simulink model "OASIS"  (R2024b)
settings: Solver=ode3  StartTime=0.0  StopTime=86400  FixedStep=1  MaxStep=0.1  RelTol=1e-3
PostLoadFcn:
  | init_OASIS
InitFcn:
  | init_OASIS
values from neighbouring files (symbols this model uses):
  DiscreteON = 1    [init_OASIS.m]
  GridON = 1    [init_OASIS.m]
  P_cargador_EV = 50000    [init_OASIS.m]
undefined symbols (not defined in the file or in its folder): DiscIntNeverNeededParam, Tamb
(part 1 of 3)
settings Model: PacingRate=0.500000  Creator=Miguel A. Ridao  LastModifiedBy=ferna
settings DebuggingCC: AlgebraicLoopMsg=none  UnconnectedInputMsg=warning  UnconnectedOutputMsg=warning  UnconnectedLineMsg=warning  UnderSpecifiedDimensionMsg=warning
settings ModelReferenceCC: EnableRefExpFcnMdlSchedulingChecks=on
settings RTWCC: GPUComputeCapability=3.5  DLArmComputeVersion=19.05

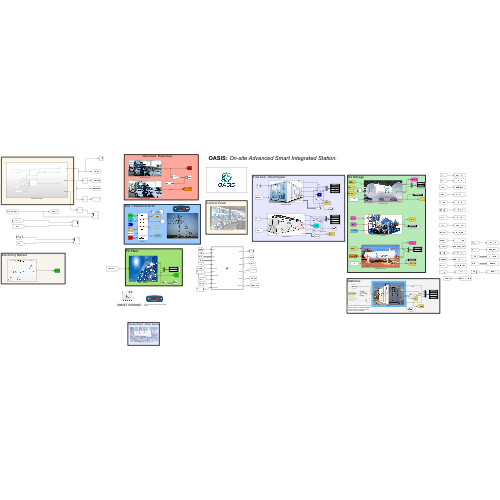
[thumbnail: Simulink's stored preview of the top-level diagram]
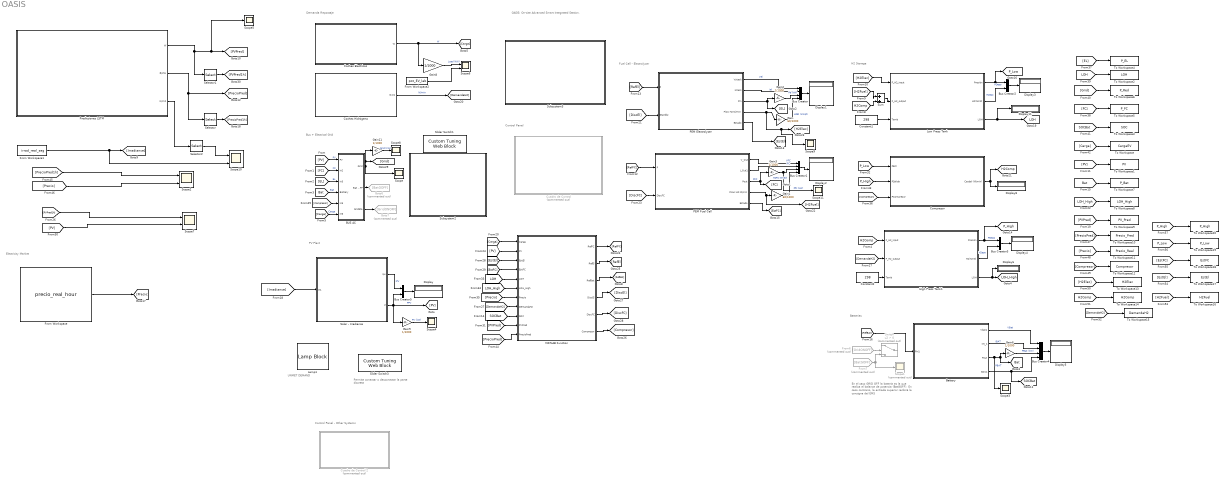
== system OASIS ==
  note: H2 Storage
  note: OASIS: On-site Advanced Smart Integrated Station.
  note: Control Panel - Other Systems
  note: En el caso GRID OFF la batería es la que realiza el balance de potencia (BatGOFF).
      | En caso contrario, la entrada superior recibirá la consigna del EMS
  note: Control Panel
  note: PV Plant
  note: Bus + Electrical Grid
  note: Demanda Repostaje
  note: Batteries
  note: Fuel Cell - Electrolyzer
  note: UNMET DEMAND
  note: Permite conectar o desconectar la parte discreta
  note: Electricity Market
  BUS AC : Subsystem
      mask Display:
      | image('Imagenes\BusAC.jpg')
      | color('red')
      | port_label('output', 1, 'Red (W)')
      | port_label('output', 2, 'Bat Grid OFF (W)')
      | port_label('output', 3, 'Grid Status')
  Battery : Subsystem  mask{Vbt0=380, CMWh=1, Kbt=0.000739, Abt=20.314, Bbt=0.00171, R=0.00027, Imax=1300, SOCact=70}
      mask prompts: Vbt0 "Open Circuit Battery Voltage, "Vbt,0" (V)"; CMWh "Maximum Capacity of the battery, "MWh)"; Kbt "Polarization Constant, "Kbt" (V)"; Abt "Amplitude of the exponential zone, "Abt" (V)"; Bbt "Inverse of the time constant in the exponencial zona, "Bbt" (A·h-1)"; R "Internal Resistance, "R" (ohms)"; Imax "Charge/Discharge Max. Current"; SOCact "SOC Initial Batteries (%)"
      mask init:
      | C120bt=CMWh*1000*1000/Vbt0
      mask DialogControl DescGroupVar Prompt: Stationary Battery model
      mask Display:
      | image('Hydor_bat.jpg')
      | color('red')
      | port_label('output', 1, 'Vbat')
      | 
      | port_label('output', 2, 'Ibat')
      | port_label('output', 3, 'Pout')
      | port_label('output', 4, 'SOC')
      | port_label('input', 1, 'P')
  Bus Creator : BusCreator  Inputs=4
  Bus Creator1 : BusCreator  Inputs=4
  Bus Creator2 : BusCreator  Inputs=2
  Bus Creator3 : BusCreator  Inputs=2
  Bus Creator4 : BusCreator  Inputs=4
  Bus Creator5 : BusCreator  Inputs=2
  Coches Electricos : Subsystem
      mask Display: image('Electric-Car.png');
  Coches Hidrógeno : Subsystem
      mask Display: image('Hydrogen_Car.png');
  Compresor : Subsystem  mask{Eficiencia=0.8, PMax=15}
      mask prompts: PMax "Potencia Máxima (kW)"
      mask Display:
      | image('Compresor.jpg'); % Use "Edit Image" on toolstrip to change.
      | color('red')
      | port_label('input', 1, 'Input Pressure [bar]')
      | port_label('input', 2, 'Output Pressure [bar]')
      | port_label('input', 3, 'Power (W)')
      | port_label('output', 1, 'H2 Flow [Nl/min]')
  Constant1 : Constant  Value=298
  Constant2 : Constant  Value=298
  Cuadro de Control : Subsystem  Commented=on
      mask Display: image('Imagenes\SCADA.jpeg')
  Cuadro de Control 2 : Subsystem  Commented=on
      mask Display: image('SCADA2.jpg'); % Use "Edit Image" on toolstrip to change.
  Display{,1..6,8,11} (9 alike) : Display
  From Workspace : FromWorkspace  VariableName=precio_real_hour  SampleTime=1  Interpolate=off  OutputAfterFinalValue=Holding final value
      mask init:
      | load('precio_horario.mat')
      mask Display: image('Imagenes\Price.PNG'); % Use "Edit Image" on toolstrip to change.
  From Workspace1 : FromWorkspace  VariableName=irrad_real_seg  SampleTime=1
  From Workspace2 : FromWorkspace  VariableName=pot_EV_lab
  From6 : From  Commented=on  GotoTag=GridONOFF
  From7 : From  Commented=on  GotoTag=BatGOFF
  Gain : Gain  Gain=60/1000
  Gain1 : Gain  Gain=60/1000
  Gain{2..3,6,8..9,11} (6 alike) : Gain  Gain=1/1000
  Goto6 : Goto  Commented=on  GotoTag=BatGOFF
  Goto7 : Goto  Commented=on  GotoTag=GridONOFF
  High Press Tank1 : Subsystem  mask{Vol=0.41, PMax=600, PIni=480}
      mask prompts: Vol "Capacidad (m3)"; PMax "Presión Máxima"; PIni "Presión Incial (bar)"
      mask Display:
      | image('Imagenes\H2DepoAlta.jpg')
      | color('red')
      | port_label('output', 1, 'Pressure [bar]')
      | port_label('output', 2, 'H2 [Nm3]')
      | port_label('output', 3, 'LOH [%]')
      | port_label('input', 1, 'H2 Elect [Nl/min]')
      | port_label('input', 2, 'H2 FC [Nl/min]')
      | port_label('input', 3, 'Temp Amb [K]')
  Lamp1 : LampBlock  LabelPosition=Hide
  Low Press Tank : Subsystem  mask{Vol=3.1, PMax=40, PIni=26}
      mask prompts: Vol "Capacidad (m3)"; PMax "Presión Máxima"; PIni "Presión Incial (bar)"
      mask Display:
      | image('Imagenes\Deposito.jpg')
      | color('red')
      | port_label('output', 1, 'Pressure [bar]')
      | port_label('output', 2, 'H2 [Nm3]')
      | port_label('output', 3, 'LOH [%]')
      | port_label('input', 1, 'H2 Elect [Nl/min]')
      | port_label('input', 2, 'H2 FC [Nl/min]')
      | port_label('input', 3, 'Temp Amb [K]')
  MATLAB Function : MATLAB Function  TreatAsAtomicUnit=on
  PEM Electrolyser : Subsystem  mask{E0=1.23, K1n=-0.9e-3, Ph2=40, Po2=1.3, Ael=1500, Rohm=1.7008e-04, iao=1.0631e-6, ico=1e-3, N=60, Tel=298, Pmax=200000, Pout=40, efc=0.7, efcv=0.97}
      mask prompts: E0 "E0 (V)"; Ph2 "Hydrogen Partial Pressure (bar)"; Po2 "Oxygen Partial Pressure (bar)"; Ael "Stack Area (cm^2)"; iao "Anode Current Density (A/cm^2)"; ico "Cathode Current Density (A/cm^2)"; N "Number of Cells in the Stack"; Tel "Electrolizer Temperature (K)"; Pmax "Max Input Power (W)"; Pout "Tank pressure (bar)"; efc "Compressor Efficiency"; efcv "Converter Efficiancy"
      mask init:
      | R=8.314472;
      | F=96485;
      | CpH2=20.79;
      | gamma=1.4;
      | 
      | ModoManual=1;
      | PElecMan=100;
      mask Help:
      | INPUTS
      | - Power (W)  Power hss to be negative
      | 
      | OUTPUTS
      | - Electrolizer Voltage (V)
      | - Electrolizar Current (I)
      | - H2 Flow (g/s)
      mask DialogControl DescGroupVar Prompt: PEM Electrolyser Model
      mask DialogControl DescTextVar Prompt: (Add text here)
      mask DialogControl ParameterGroupVar Prompt: PEM Electrolyser Parameters
      mask Display:
      | image('Hydor_elec.jpg')
      | color('red')
      | port_label('output', 1, 'Vel')
      | port_label('output', 2, 'Iel')
      | port_label('output', 4, 'H2 (Nl/min)')
      | port_label('output', 5, 'Estado')
      | port_label('output', 3, 'Pin')
      | port_label('input', 1, 'P')
  PEM Fuel Cell : Subsystem  mask{u0=0.93, K1t=0.00293, K1act=0.066098, K2act=0.012705, Rohm=0.29179, K1conc=0.028396, K2conc=8.0011, Tst=296, T0st=296, Afc=600, n=120, Imax=600}
      mask prompts: Tst "Stack Temperature (K)"; T0st "Nominal Stack Temperature (K)"; Afc "Effective Area of the Membrane (cm^2)"; n "Number of Cell in the Fuel Cell"; Imax "Max Corrent (A)"
      mask init:
      | R=8.314472;
      | F=96485;
      mask DialogControl DescGroupVar Prompt: Fuell Cell Model
      mask DialogControl ParameterGroupVar Prompt: Equation Parameters
      mask DialogControl Container4 Prompt: Fuel Cell Parameters
      mask Display:
      | image('Imagenes\Hydor_FC.jpg')
      | color('red')
      | port_label('output', 1, 'Vst')
      | 
      | 
      | port_label('input', 1, 'P')
      | 
      | port_label('output', 3, 'Pout')
      | 
      | port_label('output', 2, 'Ist')
      | port_label('output', 4, 'H2 (Nl/min)')
      | port_label('output', 5, 'Estado')
  Predicciones LSTM : Subsystem
  Scope{,3..5,8..9,11} (7 alike) : Scope
  Scope1 : Scope  Commented=on
  Scope{2,6..7,10} (4 alike) : Scope  NumInputPorts=2
  Selector : Selector  InputPortWidth=24  IndexOptions=Index vector (dialog)  Indices=[1]  OutputSizes=1
  Selector1 : Selector  InputPortWidth=24  IndexOptions=Index vector (dialog)  Indices=[1]  OutputSizes=1
  Selector2 : Selector  InputPortWidth=24  IndexOptions=Index vector (dialog)  Indices=[1]  OutputSizes=1
  Slider Switch1 : CustomTuningWebBlock  LabelPosition=Hide  ShowInitialText=on  Configuration="{\"components\":[{\"name\":\"CustomSwitchStateComponent\",\"settings\":{\"position\":[0,0,1,1],\"states\":[{\"HitRegion\":{\"position\":[0,0,0.5,1]},\"Image\":{\"position\":[0,0,1,1],\"size\":[1,1],\"src\":\"data:image\\/svg+xml;base64,PD94bWwgdmVyc2lvbj0iMS4wIiBlbmNvZGluZz0idXRmLTgiPz4NCjwhLS0gR2VuZXJhdG9yOiBBZG9iZSBJbGx1c3RyYXRvciAyNS4yLjEsIFNWRyBFeHBvcnQgUGx1Zy1JbiAuIFNWRyBWZXJzaW9uOiA2LjAwIEJ1aWxkIDApICAtLT4NCjxzdmcgdmVyc2lvbj0iMS4xIiB4bWxucz0iaHR0cDovL3d3dy53My5vcmcvMjAwMC9zdmciIHhtbG5zOnhsaW5rPSJodHRwOi8vd3d3LnczLm9yZy8xOTk5L3hsaW5rIiB4PSIwcHgiIHk9IjBweCINCgkgdmlld0JveD0iMCAwIDc2IDI5IiBzdHlsZT0iZW5hYmxlLWJhY2tncm91bmQ6bmV3 ...(+5404 chars)\",\"srcOrientation\":\"Right\"},\"Label\":{\"color\":[0.9882352941176471,0.9882352941176471,0.7725490196078432],\"icon\":{\"size\":[0,0],\"src\":[],\"srcOrientation\":\"Right\"},\"iconPlacement\":\"left\",\"opacity\":1,\"position\":[0.5,0.14],\"show\":true,\"text\":{\"content\":\"Off\",\"font\":\"Helvetica\"}},\"Value\":0},{\"HitRegion\":{\"position\":[0,0.5,0.5,1]},\"Image\":{\"position\":[0,0,1,1],\"size\":[1,1],\"src\":\"data:image\\/svg+xml;base64,PD94bWwgdmVyc2lvbj0iMS4wIiBlbmNvZGluZz0idXRmLTgiPz4NCjwhLS0gR2VuZXJhdG9yOiBBZG9iZSBJbGx1c3RyYXRvciAyNS4yLjEsIFNWRyBFeHBvcnQgUGx1Zy1JbiAuIFNWRyBWZXJzaW9uOiA2LjAwIEJ1aWxkIDApICAtLT4NCjxzdmcgdmVyc2lvbj0iMS4xIiB4bWxucz0iaHR0cDovL3d3dy53My5vcmcvMjAwMC9zdmciIHhtbG5zOnhsaW5rPSJodHRwOi8vd3d3LnczLm9yZy8xOTk5L3hsaW5rIiB4PSIwcHgiIHk9IjBweCINCgkgdmlld0JveD0iMCAwIDc2IDI5IiBzdHlsZT0iZW5hYmxlLWJhY2tncm91bmQ6bmV3 ...(+5404 chars)\",\"srcOrientation\":\"Right\"},\"Label\":{\"color\":[0.9882352941176471,0.9882352941176471,0.7725490196078432],\"icon\":{\"size\":[0,0],\"src\":[],\"srcOrientation\":\"Right\"},\"iconPlacement\":\"left\",\"opacity\":1,\"position\":[0.5,0.86],\"show\":true,\"text\":{\"content\":\"On\",\"font\":\"Helvetica\"}},\"Value\":1}]}},{\"name\":\"BackgroundImageComponent\",\"settings\":{\"image\":{\"size\":[0,0],\"src\":\"default\",\"srcOrientation\":[]},\"position\":[0,0,1,1],\"scaleMode\":\"0\"}},{\"name\":\"ForegroundImageComponent\",\"settings\":{\"image\":{\"size\":[0,0],\"src\":\"default\",\"srcOrientation\":[]},\"isForeground\":1,\"position\":[0,0,1,1],\"scaleMode\":\"0\"}}],\"settings\":{\"BindingType\":\"param\",\"backgroundColor\":[0,0,255,\"1\"],\"fixedAspectRatio\":\"on\",\"foregroundColor\":[234,234,234],\"showBackgroundColor\":false,\"variant\":\"slider\",\"version\":\"R2024b\"},\"type\":\"Switch\"}"
  Slider Switch3 : CustomTuningWebBlock  LabelPosition=Hide  ShowInitialText=on  Configuration="{\"components\":[{\"name\":\"CustomSwitchStateComponent\",\"settings\":{\"position\":[0,0,1,1],\"states\":[{\"HitRegion\":{\"position\":[0,0,0.5,1]},\"Image\":{\"position\":[0,0,1,1],\"size\":[1,1],\"src\":\"data:image\\/svg+xml;base64,PD94bWwgdmVyc2lvbj0iMS4wIiBlbmNvZGluZz0idXRmLTgiPz4NCjwhLS0gR2VuZXJhdG9yOiBBZG9iZSBJbGx1c3RyYXRvciAyNS4yLjEsIFNWRyBFeHBvcnQgUGx1Zy1JbiAuIFNWRyBWZXJzaW9uOiA2LjAwIEJ1aWxkIDApICAtLT4NCjxzdmcgdmVyc2lvbj0iMS4xIiB4bWxucz0iaHR0cDovL3d3dy53My5vcmcvMjAwMC9zdmciIHhtbG5zOnhsaW5rPSJodHRwOi8vd3d3LnczLm9yZy8xOTk5L3hsaW5rIiB4PSIwcHgiIHk9IjBweCINCgkgdmlld0JveD0iMCAwIDc2IDI5IiBzdHlsZT0iZW5hYmxlLWJhY2tncm91bmQ6bmV3 ...(+5404 chars)\",\"srcOrientation\":\"Right\"},\"Label\":{\"color\":[0.9882352941176471,0.9882352941176471,0.7725490196078432],\"icon\":{\"size\":[0,0],\"src\":[],\"srcOrientation\":\"Right\"},\"iconPlacement\":\"left\",\"opacity\":1,\"position\":[0.5,0.14],\"show\":true,\"text\":{\"content\":\"Off\",\"font\":\"Helvetica\"}},\"Value\":0},{\"HitRegion\":{\"position\":[0,0.5,0.5,1]},\"Image\":{\"position\":[0,0,1,1],\"size\":[1,1],\"src\":\"data:image\\/svg+xml;base64,PD94bWwgdmVyc2lvbj0iMS4wIiBlbmNvZGluZz0idXRmLTgiPz4NCjwhLS0gR2VuZXJhdG9yOiBBZG9iZSBJbGx1c3RyYXRvciAyNS4yLjEsIFNWRyBFeHBvcnQgUGx1Zy1JbiAuIFNWRyBWZXJzaW9uOiA2LjAwIEJ1aWxkIDApICAtLT4NCjxzdmcgdmVyc2lvbj0iMS4xIiB4bWxucz0iaHR0cDovL3d3dy53My5vcmcvMjAwMC9zdmciIHhtbG5zOnhsaW5rPSJodHRwOi8vd3d3LnczLm9yZy8xOTk5L3hsaW5rIiB4PSIwcHgiIHk9IjBweCINCgkgdmlld0JveD0iMCAwIDc2IDI5IiBzdHlsZT0iZW5hYmxlLWJhY2tncm91bmQ6bmV3 ...(+5404 chars)\",\"srcOrientation\":\"Right\"},\"Label\":{\"color\":[0.9882352941176471,0.9882352941176471,0.7725490196078432],\"icon\":{\"size\":[0,0],\"src\":[],\"srcOrientation\":\"Right\"},\"iconPlacement\":\"left\",\"opacity\":1,\"position\":[0.5,0.86],\"show\":true,\"text\":{\"content\":\"On\",\"font\":\"Helvetica\"}},\"Value\":1}]}},{\"name\":\"BackgroundImageComponent\",\"settings\":{\"image\":{\"size\":[0,0],\"src\":\"default\",\"srcOrientation\":[]},\"position\":[0,0,1,1],\"scaleMode\":\"0\"}},{\"name\":\"ForegroundImageComponent\",\"settings\":{\"image\":{\"size\":[0,0],\"src\":\"default\",\"srcOrientation\":[]},\"isForeground\":1,\"position\":[0,0,1,1],\"scaleMode\":\"0\"}}],\"settings\":{\"BindingType\":\"param\",\"backgroundColor\":[0,0,255,\"1\"],\"fixedAspectRatio\":\"on\",\"foregroundColor\":[234,234,234],\"showBackgroundColor\":false,\"variant\":\"slider\",\"version\":\"R2024b\"},\"type\":\"Switch\"}"
  Solar - Irradiance : Subsystem  mask{npar=35, nser=24, Vp=34.60, Isc=18.57, Voc=41.7, Tc=300}
      mask prompts: npar "Number of modules in parallel"; nser "Number of modules in serie"; Vp "Voltage in the Maximun Power Point (V)"; Isc "Short Circuit Current (A)"; Voc "Open circuit Voltage (V)"; Tc "Temperature (K)"
      mask init:
      | % electron charge
      | e=1.6e-19;%(C)
      | %Boltzman constant
      | k=1.381e-23;%(J/K)
      | %Serial Resistor
      | Rs=0.1;
      mask DialogControl DescGroupVar Prompt: Photovoltaic Cell Model
      mask Display:
      | image('Imagenes\sun.jpg')
      | color('red')
      | port_label('output', 1, 'Ipv')
      | port_label('output', 2, 'Psf')
  Subsystem2 : Subsystem
      mask Display: image('Red.jpeg'); % Use "Edit Image" on toolstrip to change.
  Subsystem3 : Subsystem
      mask Display: image('OASIS.png');
  Sum : Sum  Inputs=|++
  Switch : Switch  Commented=on  Criteria=u2 > Threshold  SaturateOnIntegerOverflow=off  InputSameDT=off
  To Workspace : ToWorkspace  VariableName=CargaEV  SaveFormat=Timeseries  SampleTime=-1
  To Workspace1 : ToWorkspace  VariableName=PV  SaveFormat=Timeseries  SampleTime=-1
  To Workspace10 : ToWorkspace  VariableName=Precio_Pred  SaveFormat=Timeseries  SampleTime=-1
  To Workspace11 : ToWorkspace  VariableName=Precio_Real  SaveFormat=Timeseries  SampleTime=-1
  To Workspace12 : ToWorkspace  VariableName=Compresor  SaveFormat=Timeseries  SampleTime=-1
  To Workspace13 : ToWorkspace  VariableName=H2Elec  SaveFormat=Timeseries  SampleTime=-1
  To Workspace14 : ToWorkspace  VariableName=H2Comp  SaveFormat=Timeseries  SampleTime=-1
  To Workspace15 : ToWorkspace  VariableName=DemandaH2  SaveFormat=Timeseries  SampleTime=-1
  To Workspace16 : ToWorkspace  VariableName=H2Fuel  SaveFormat=Timeseries  SampleTime=-1
  To Workspace17 : ToWorkspace  VariableName=EstEl  SaveFormat=Timeseries  SampleTime=-1
  To Workspace18 : ToWorkspace  VariableName=EstFC  SaveFormat=Timeseries  SampleTime=-1
  To Workspace19 : ToWorkspace  VariableName=P_Low  SaveFormat=Timeseries  SampleTime=-1
  To Workspace2 : ToWorkspace  VariableName=LOH  SaveFormat=Timeseries  SampleTime=-1
  To Workspace20 : ToWorkspace  VariableName=P_High  SaveFormat=Timeseries  SampleTime=-1
  To Workspace3 : ToWorkspace  VariableName=SOC  SaveFormat=Timeseries  SampleTime=-1
  To Workspace4 : ToWorkspace  VariableName=P_EL  SaveFormat=Timeseries  SampleTime=-1
  To Workspace5 : ToWorkspace  VariableName=P_FC  SaveFormat=Timeseries  SampleTime=-1
  To Workspace6 : ToWorkspace  VariableName=P_Red  SaveFormat=Timeseries  SampleTime=-1
  To Workspace7 : ToWorkspace  VariableName=P_Bat  SaveFormat=Timeseries  SampleTime=-1
  To Workspace8 : ToWorkspace  VariableName=LOH_High  SaveFormat=Timeseries  SampleTime=-1
  To Workspace9 : ToWorkspace  VariableName=PV_Pred  SaveFormat=Timeseries  SampleTime=-1
  tag scope: Bat=global, H2Comp=global, LOH=global, LOH_High=global, P_High=global, P_Low=global, SOCBat=global
  wires:
  Solar - Irradiance/1(Ipv) -> Bus Creator5/1  "IPV"
  PEM Electrolyser/1(Vstack) -> Bus Creator/1  "Vel"
  PEM Electrolyser/2(Istack) -> Bus Creator/2  "Iel"
  PEM Electrolyser/3(Pin) -> Gain2/1, [EL]
  PEM Electrolyser/4("Flow H2 Nl/min ") -> Scope9/1, [H2Elec], Gain/1
  Low Press Tank/1(Presión) -> [P_Low], Bus Creator2/1  "PDepo"
  Low Press Tank/2(H2(Nm3)) -> Bus Creator2/2  "H2epo"
  Constant1/1 -> Low Press Tank/3(Tamb)
  Gain/1 -> Bus Creator/4  "H2El  Nm3/h"
  PEM Fuel Cell/1(V_Out) -> Bus Creator1/1  "VFC"
  PEM Fuel Cell/3(Pout) -> Gain3/1, [FC]  "PFC"
  PEM Fuel Cell/4(Flowl H2 Nl/min) -> [H2Fuel], Gain1/1
  Gain1/1 -> Bus Creator1/4  "H2FC Nm3/h"
  Battery/2(Int_1) -> Bus Creator4/2  "IBAT"
  Battery/4(SOC1) -> [SOCBat], Bus Creator4/4
  Coches Electricos/1(W) -> Gain8/1, [Carga]  "W"
  [PV] -> BUS AC/1(PV)  "PV"
  [FC] -> BUS AC/2(In2)  "FC"
  [EL] -> BUS AC/3(In3)  "EL"
  [Bat] -> BUS AC/4(Battery)  "Bat"
  [Carga] -> BUS AC/6(In6)  "Carga"
  PEM Fuel Cell/2(I_Out1) -> Bus Creator1/2  "IFC"
  Bus Creator/1 -> Display1/1
  Gain2/1 -> Bus Creator/3  "Pe (kW)"
  Bus Creator1/1 -> Display2/1
  Bus Creator2/1 -> Display3/1
  Battery/1(Vbat1) -> Bus Creator4/1  "VBat"
  Battery/3(Pout) -> Scope3/1, Gain6/1, [Bat]  "PBAT"
  Bus Creator4/1 -> Display5/1
  Solar - Irradiance/2(P) -> [PV], Gain9/1, Bus Creator5/2  "PPV"
  Bus Creator5/1 -> Display/1
  Gain3/1 -> Scope11/1, Bus Creator1/3  "Pfc (kW)"
  BUS AC/1(Grid) -> Scope/1, Gain11/1, [Grid]
  BUS AC/2(Bat GOFF) -> Goto6/1
  BUS AC/3(GridSta) -> Goto7/1
  From6/1 -> Switch/2
  From7/1 -> Scope1/1, Switch/3
  Gain6/1 -> Bus Creator4/3  "PBat (kW)"
  [RefFC] -> PEM Fuel Cell/1(P)
  [RefEl] -> PEM Electrolyser/1(P)
  Gain8/1 -> Scope6/1  "Load (kW)"
  Gain9/1 -> Scope4/1  "PV (kW)"
  Gain11/1 -> Scope8/1  "Grid (kW)"
  PEM Electrolyser/5(Estado) -> [EstEl]
  [DiscEl] -> PEM Electrolyser/2(Standby)
  PEM Fuel Cell/5(Estado) -> [EstFC]
  [DiscFC] -> PEM Fuel Cell/2(DiscFC)
  Low Press Tank/3(LOH) -> Display11/1, [LOH]
  [RefBat] -> Battery/1(Pin1)
  Constant2/1 -> High Press Tank1/3(Tamb)
  High Press Tank1/3(LOH) -> Display6/1, [LOH_High]
  Bus Creator3/1 -> Display4/1
  High Press Tank1/1(Presión) -> [P_High], Bus Creator3/1  "PDepo"
  High Press Tank1/2(H2(Nm3)) -> Bus Creator3/2  "H2epo"
  [P_Low] -> Compresor/1(PEnt)
  [P_High] -> Compresor/2(PSalida)
  Compresor/1(Caudal (Nl/min)) -> [H2Comp], Display8/1
  [H2Comp] -> High Press Tank1/1(F_H2_input)
  Sum/1 -> Low Press Tank/2(F_H2_output)
  [H2Fuel] -> Sum/1
  [H2Comp] -> Sum/2
  [H2Elec] -> Low Press Tank/1(F_H2_input)
  [DemandaH2] -> High Press Tank1/2(F_H2_output)
  [Carga] -> MATLAB Function/1(Carga)
  [PV] -> MATLAB Function/2(PV)
  [EstEl] -> MATLAB Function/3(EstEl)
  [EstFC] -> MATLAB Function/4(EstFC)
  [LOH] -> MATLAB Function/5(LOH)
  [LOH_High] -> MATLAB Function/6(LOH_High)
  [Precio] -> MATLAB Function/7(Precio)
  MATLAB Function/1(RefFC) -> [RefFC]
  MATLAB Function/2(RefEl) -> [RefEl]
  MATLAB Function/4(DiscEl) -> [DiscEl]
  MATLAB Function/5(DiscFC) -> [DiscFC]
  [DemandaH2] -> MATLAB Function/8(DemandaH2)
  [Compresor] -> Compresor/3(PCompresor)
  MATLAB Function/6(Compresor) -> [Compresor]
  Coches Hidrógeno/1(Out1) -> [DemandaH2]  "Nl/min"
  [EL] -> To Workspace4/1
  [FC] -> To Workspace5/1
  [LOH] -> To Workspace2/1
  [Grid] -> To Workspace6/1
  [SOCBat] -> To Workspace3/1
  [Carga] -> To Workspace/1
  [PV] -> To Workspace1/1
  [SOCBat] -> MATLAB Function/9(SOC)
  MATLAB Function/3(RefBat) -> [RefBat]
  [Bat] -> To Workspace7/1
  [LOH_High] -> To Workspace8/1
  [Compresor] -> BUS AC/5(In5)
  From Workspace1/1 -> Scope10/2, [Irradiance]
  [Irradiance] -> Solar - Irradiance/1(In1)
  [PVPred] -> To Workspace9/1
  [PV] -> Scope7/2
  [PVPred1h] -> Scope7/1
  [PVPred] -> MATLAB Function/10(PVPred)
  From Workspace/1 -> [Precio]
  Predicciones LSTM/1(W) -> Selector1/1, Scope5/1, [PVPred]
  Predicciones LSTM/2(€/MW) -> Selector/1, [PrecioPred]
  [Precio] -> Scope2/2
  [PrecioPred1h] -> Scope2/1
  Selector/1 -> [PrecioPred1h]
  Selector1/1 -> [PVPred1h]
  [PrecioPred] -> MATLAB Function/11(PrecioPred)
  Predicciones LSTM/3(W/m2) -> Selector2/1
  Selector2/1 -> Scope10/1
  [PrecioPred] -> To Workspace10/1
  [Precio] -> To Workspace11/1
  From Workspace2/1 -> Scope6/2
  [Compresor] -> To Workspace12/1
  [H2Elec] -> To Workspace13/1
  [H2Comp] -> To Workspace14/1
  [DemandaH2] -> To Workspace15/1
  [H2Fuel] -> To Workspace16/1
  [EstEl] -> To Workspace17/1
  [EstFC] -> To Workspace18/1
  [P_Low] -> To Workspace19/1
  [P_High] -> To Workspace20/1

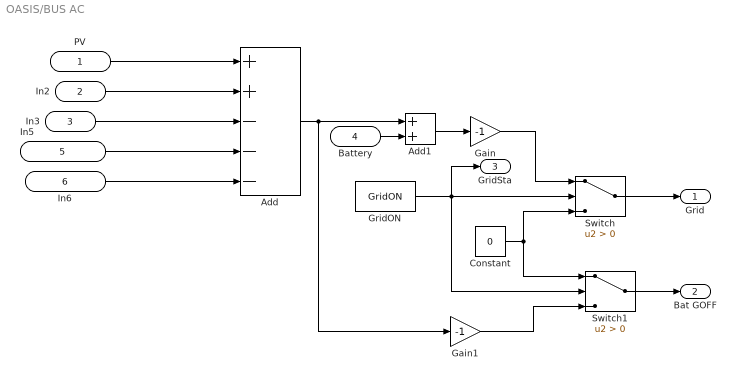
== system OASIS/BUS AC ==
  PV : Inport
  In2 : Inport  Port=2
  In3 : Inport  Port=3
  Battery : Inport  Port=4
  In5 : Inport  Port=5
  In6 : Inport  Port=6
  Add : Sum  Inputs=++---
  Add1 : Sum
  Constant : Constant  Value=0
  Gain : Gain  Gain=-1
  Gain1 : Gain  Gain=-1
  GridON : Constant  Value=GridON
  Switch : Switch  Criteria=u2 > Threshold  SaturateOnIntegerOverflow=off  InputSameDT=off
  Switch1 : Switch  Criteria=u2 > Threshold  SaturateOnIntegerOverflow=off  InputSameDT=off
  Grid : Outport
  Bat GOFF : Outport  Port=2
  GridSta : Outport  Port=3
  wires:
  GridON/1 -> GridSta/1, Switch/2, Switch1/2
  PV/1 -> Add/1
  In2/1 -> Add/2
  In3/1 -> Add/3
  In6/1 -> Add/5
  Add/1 -> Gain1/1, Add1/1
  Battery/1 -> Add1/2
  Add1/1 -> Gain/1
  Gain/1 -> Switch/1
  Switch/1 -> Grid/1
  Constant/1 -> Switch/3, Switch1/1
  Switch1/1 -> Bat GOFF/1
  Gain1/1 -> Switch1/3
  In5/1 -> Add/4

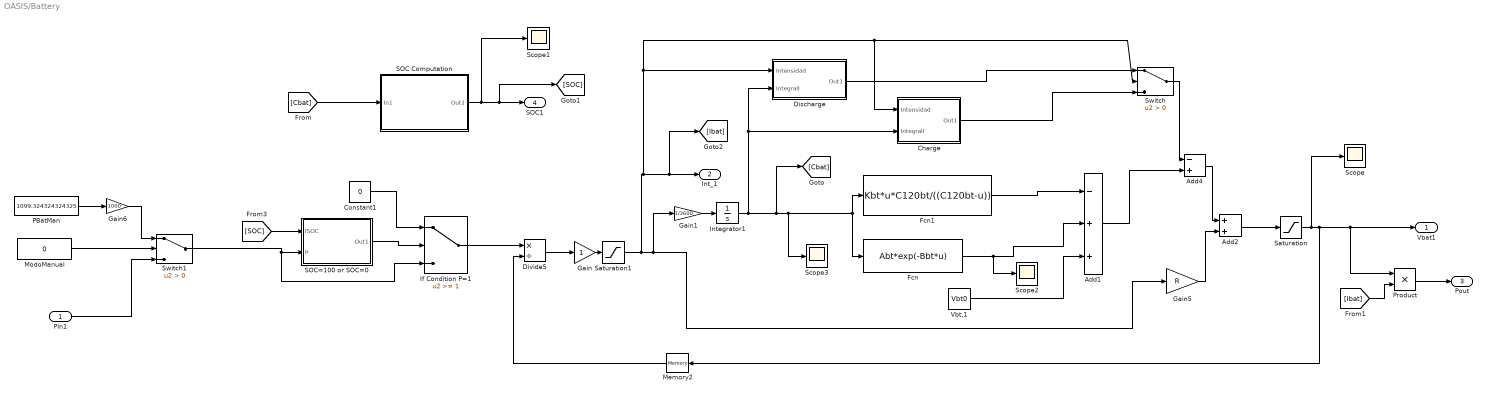
== system OASIS/Battery ==
  Pin1 : Inport
  Add1 : Sum  Inputs=-++
  Add2 : Sum
  Add4 : Sum  Inputs=-+
  Charge : Subsystem
  Constant1 : Constant  Value=0
  Discharge : Subsystem
  Divide5 : Product  Inputs=*/
  Fcn : Fcn  Expr=Abt*exp(-Bbt*u)
  Fcn1 : Fcn  Expr=Kbt*u*C120bt/((C120bt-u))
  Gain : Gain
  Gain1 : Gain  Gain=1/3600
  Gain5 : Gain  Gain=R
  Gain6 : Gain  Gain=1000
  If Condition P=1 : Switch  Threshold=1  SaturateOnIntegerOverflow=off  InputSameDT=off
  Integrator1 : Integrator  InitialCondition=C120bt-(SOCact/100)*C120bt  LimitOutput=on  UpperSaturationLimit=C120bt  LowerSaturationLimit=0
  Memory2 : Memory  InitialCondition=48
  ModoManual : Constant  Value=0
  PBatMan : Constant  Value=1099.324324324325
  Product : Product
  SOC Computation : Subsystem
  SOC=100 or SOC=0 : Subsystem
  Saturation : Saturate  UpperLimit=inf  LowerLimit=1
  Saturation1 : Saturate  UpperLimit=Imax  LowerLimit=-Imax
  Scope{,1..3} (4 alike) : Scope
  Switch : Switch  Criteria=u2 > Threshold  SaturateOnIntegerOverflow=off  InputSameDT=off
  Switch1 : Switch  Criteria=u2 > Threshold  SaturateOnIntegerOverflow=off  InputSameDT=off
  Vbt,1 : Constant  Value=Vbt0
  Vbat1 : Outport  VectorParamsAs1DForOutWhenUnconnected=off
  Int_1 : Outport  Port=2  VectorParamsAs1DForOutWhenUnconnected=off
  Pout : Outport  Port=3  VectorParamsAs1DForOutWhenUnconnected=off
  SOC1 : Outport  Port=4  VectorParamsAs1DForOutWhenUnconnected=off
  wires:
  ModoManual/1 -> Switch1/2
  Pin1/1 -> Switch1/3
  Gain6/1 -> Switch1/1
  PBatMan/1 -> Gain6/1
  [Ibat] -> Product/2
  SOC=100 or SOC=0/1(Out1) -> If Condition P=1/2
  [Cbat] -> SOC Computation/1(In1)
  Saturation/1 -> Scope/1, Memory2/1, Vbat1/1, Product/1
  Integrator1/1 -> Charge/2(IntegralI), Discharge/2(IntegralI), Scope3/1, Fcn/1, Fcn1/1, [Cbat]
  [SOC] -> SOC=100 or SOC=0/1(ISOC)
  Product/1 -> Pout/1
  Gain/1 -> Saturation1/1
  Discharge/1(Out1) -> Switch/1
  Add4/1 -> Add2/1
  Memory2/1 -> Divide5/2
  Constant1/1 -> If Condition P=1/1
  Fcn1/1 -> Add1/1
  Switch/1 -> Add4/1
  Charge/1(Out1) -> Switch/3
  Saturation1/1 -> Charge/1(Intensidad), Switch/2, Discharge/1(Intensidad), [Ibat], Int_1/1, Gain1/1, Gain5/1
  If Condition P=1/1 -> Divide5/1
  Fcn/1 -> Scope2/1, Add1/2
  SOC Computation/1(Out1) -> Scope1/1, [SOC], SOC1/1
  Gain1/1 -> Integrator1/1
  Add1/1 -> Add4/2
  Vbt,1/1 -> Add1/3
  Add2/1 -> Saturation/1
  Switch1/1 -> If Condition P=1/3, SOC=100 or SOC=0/2(P)
  Gain5/1 -> Add2/2
  Divide5/1 -> Gain/1

== system OASIS/Coches Electricos ==
  Display : Display
  From Workspace : FromWorkspace  VariableName=demanda_EV  SampleTime=1  Interpolate=off  OutputAfterFinalValue=Holding final value
      mask init:
      | load('precio_horario.mat')
      mask Display: disp('Llegada de coches EV');
  Gain1 : Gain  Gain=P_cargador_EV/0.9
  Gain2 : Gain  Gain=1/3600000
  Integrator : Integrator
  W : Outport
  wires:
  Gain1/1 -> Integrator/1, W/1
  From Workspace/1 -> Gain1/1  "Nº Cargadores Activos"
  Integrator/1 -> Gain2/1
  Gain2/1 -> Display/1  "kWh"

== system OASIS/Coches Hidrógeno ==
  Display : Display
  Display1 : Display
  From Workspace : FromWorkspace  VariableName=demanda_H2  SampleTime=1  Interpolate=off  OutputAfterFinalValue=Holding final value
      mask init:
      | load('precio_horario.mat')
      mask Display: disp('Llegada de coches H2');
  Gain1 : Gain  Gain=667560
  Gain2 : Gain  Gain=57.5
  Integrator : Integrator
  Out1 : Outport
  wires:
  From Workspace/1 -> Integrator/1, Gain1/1  "kg/s"
  Gain1/1 -> Out1/1  "Nl/min"
  Gain2/1 -> Display/1  "kWh"
  Integrator/1 -> Display1/1, Gain2/1

== system OASIS/Compresor ==
  PEnt : Inport
  PSalida : Inport  Port=2
  PCompresor : Inport  Port=3
  Constant : Constant  Value=PMax
  Gain : Gain  Gain=667408
  Gain1 : Gain  Gain=Eficiencia
  Gain2 : Gain  Gain=1000
  MATLAB Function : MATLAB Function  TreatAsAtomicUnit=on
  Switch : Switch  Criteria=u2 > Threshold  Threshold=PMax*1000  SaturateOnIntegerOverflow=off  InputSameDT=off
  Caudal (Nl/min) : Outport
  wires:
  PSalida/1 -> MATLAB Function/2(PSalida)
  PEnt/1 -> MATLAB Function/1(PEnt)
  MATLAB Function/1(Caudal) -> Gain/1  "kg/s"
  Gain/1 -> Gain1/1
  Gain1/1 -> Caudal (Nl/min)/1
  PCompresor/1 -> Switch/2, Switch/3
  Constant/1 -> Gain2/1
  Gain2/1 -> Switch/1
  Switch/1 -> MATLAB Function/3(PCompresor)
